simulink model "a_zishiying_try"  (R2018a)
settings: Solver=ode23tb  StartTime=0.0  StopTime=50  RelTol=1e-3
settings Model: Creator=lenovo  LastModifiedBy=lenovo

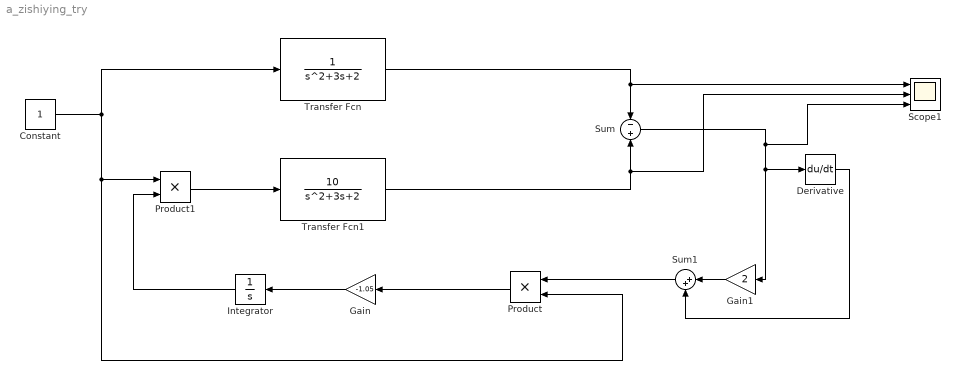
== system a_zishiying_try ==
  Constant : Constant
  Derivative : Derivative
  Gain : Gain  Gain=-1.05
  Gain1 : Gain  Gain=2
  Integrator : Integrator
  Product : Product
  Product1 : Product
  Scope1 : Scope  NumInputPorts=3
  Sum : Sum  Inputs=-|+
  Sum1 : Sum  Inputs=|++
  Transfer Fcn : TransferFcn  Denominator=[1 3 2]
  Transfer Fcn1 : TransferFcn  Numerator=[10]  Denominator=[1 3 2]
  wires:
  Transfer Fcn/1 -> Sum/1, Scope1/1
  Transfer Fcn1/1 -> Scope1/2, Sum/2
  Constant/1 -> Product1/1, Product/2, Transfer Fcn/1
  Gain/1 -> Integrator/1
  Product/1 -> Gain/1
  Sum/1 -> Scope1/3, Derivative/1, Gain1/1
  Sum1/1 -> Product/1
  Derivative/1 -> Sum1/2
  Gain1/1 -> Sum1/1
  Product1/1 -> Transfer Fcn1/1
  Integrator/1 -> Product1/2
